simulink model "IEEE24bus"  (R2019b)
settings: Solver=VariableStepAuto  StartTime=0.0  StopTime=100  RelTol=1e-3
values from neighbouring files (symbols this model uses):
  C_b = 1/(w_b*Z_b)    (= 5.01433343075e-06)    [IEEE24_bus.m]
  Exc = [ 011	0	 200	0.02	1.12   0.5   0	0       0       0       0       0 ... (first row only)    [IEEE24_bus.m]
  G_data = [ 011	15.8 138	2.8	0.2     2.7	1.5     0.3     7.5     0.25	0.04	0.85	0.85	0.25	0.12	0 ... (first row only)    [IEEE24_bus.m]
  H011 = 4    [IEEE24_bus.m]
  H012 = 4    [IEEE24_bus.m]
  H013 = 4    [IEEE24_bus.m]
  H021 = 4    [IEEE24_bus.m]
  H022 = 4    [IEEE24_bus.m]
  H023 = 4    [IEEE24_bus.m]
  H024 = 4    [IEEE24_bus.m]
  H025 = 4    [IEEE24_bus.m]
  H026 = 4    [IEEE24_bus.m]
  H131 = 4    [IEEE24_bus.m]
  H132 = 4    [IEEE24_bus.m]
  H133 = 4    [IEEE24_bus.m]
  H134 = 4    [IEEE24_bus.m]
  H135 = 4    [IEEE24_bus.m]
  H151 = 4    [IEEE24_bus.m]
  H152 = 4    [IEEE24_bus.m]
  H153 = 4    [IEEE24_bus.m]
  H154 = 4    [IEEE24_bus.m]
  H161 = 4    [IEEE24_bus.m]
  H181 = 3.25    [IEEE24_bus.m]
  H211 = 4    [IEEE24_bus.m]
  H212 = 4    [IEEE24_bus.m]
  H213 = 4    [IEEE24_bus.m]
  H215 = 4    [IEEE24_bus.m]
  H216 = 4    [IEEE24_bus.m]
  H221 = 3.25    [IEEE24_bus.m]
  H231 = 4    [IEEE24_bus.m]
  H232 = 4    [IEEE24_bus.m]
  H233 = 4    [IEEE24_bus.m]
  H234 = 4    [IEEE24_bus.m]
  H235 = 4    [IEEE24_bus.m]
  L_b = Z_b/w_b    (= 1.40321608159)    [IEEE24_bus.m]
  PSSMODEL = 1    [IEEE24_bus.m]    (also in IEEE24bus_simplified_benchmark.m)
  Z_b = (V_b^2)/S_b    (= 529)    [IEEE24_bus.m]
undefined symbols (not defined in the file or in its folder): D1, Delta
libraries: powerlib x258, sps_avr x33, microgridLibrary x6
(part 2 of 6)

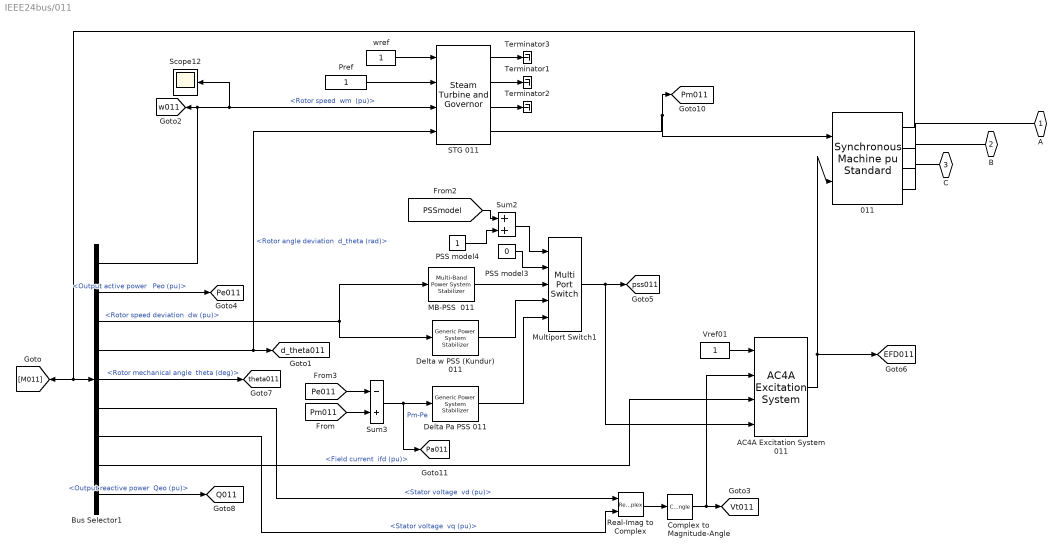
== system IEEE24bus/011 ==
  011 : powerlib/Machines/Synchronous Machine pu Standard  PresetModel=No  MechanicalLoad=Mechanical power Pm  ShowDetailedParameters=on  RotorType=Round  Units=per unit standard parameters  MeasurementBus=off  NominalParameters="[31.6*1E6  G_data(1,3)*1E3  60]"  Reactances1=[G_data(1,6),G_data(1,8),G_data(1,10),G_data(1,7),G_data(1,12),G_data(1,14),G_data(1,5)]  Reactances2=[G_data(6,6),G_data(6,8),G_data(6,10),G_data(6,7),G_data(6,12),G_data(6,14),G_data(6,5)]  dAxisTimeConstants=Open-circuit  qAxisTimeConstants=Open-circuit  TimeConstants1="[G_data(6,9)  G_data(6,11)  G_data(6,13)  G_data(6,15)]"  TimeConstants2="[G_data(1,9)  G_data(1,11)  G_data(1,13)  G_data(1,15)]"  TimeConstants3="[  5.9  0.033  0.023  ]"  TimeConstants4=[ 8.0, 0.03, 0.3371, 0.0295 ]  TimeConstants5=[ 1.01, 0.053, 0.1 ]  TimeConstants6=[ 1.3201, 0.023, 1.0, 0.07 ]  TimeConstants7="[  1.01  0.053  0.051266  ]"  TimeConstants8=[ 1.3201, 0.0231, 0.3371, 0.0295 ]  StatorResistance=0  Mechanical="[ H011 0  4 ]"  PolePairs=4  InitialConditions=[0 -49.0871 0.832503 0.832503 0.832503 -10.6328 -130.633 109.367 2.39024]  SetSaturation=off  Saturation=[0.6404,0.7127,0.8441,0.9214,0.9956,1.082,1.19,1.316,1.457;0.7,0.7698,0.8872,0.9466,0.9969,1.046,1.1,1.151,1.201]  LoadFlowParameters=[1 3330000000 20000 0 0]  TsPowergui=0  TsBlock=-1  IterativeModel=Forward Euler  IterativeDiscreteModel=Trapezoidal non iterative  BusType=PV  Pref=31.6*1e6  Qref=0  Qmin=-inf  Qmax=inf  PLF=0  QLF=0
      settings: SourceProductName=Simscape Power Systems
  AC4A Excitation System 011 : sps_avr/AC4A Excitation System  Tr=Exc(1,2)  KaTa="[Exc(1,3)   Exc(1,4)]"  VIminmax=[-10 10]  VRminmax=[-4.53 5.64]  TbTc="[Exc(1,5)  Exc(1,6)]"  Kc=0  v0=[1 2.3902]  TsBlock=0
      settings: SourceProductName=Simscape Power Systems  SourceProductBaseCode=PS
  Bus Selector1 : BusSelector  OutputSignals="Mechanical.Rotor speed  wm  (pu),Output active power   Peo (pu),Mechanical.Rotor speed deviation  dw (pu),Mechanical.Rotor angle deviation  d_theta (rad),Mechanical.Rotor mechanical angle  theta (deg),dq0 components.Stator voltage  vd (pu),dq0 components.Stator voltage  vq (pu),dq0 components.Field current  ifd (pu),Output reactive power  Qeo (pu)"
  Complex to Magnitude-Angle : ComplexToMagnitudeAngle  Output=Magnitude
  "Delta Pa PSS 011 " : powerlib/Machines/Generic Power System Stabilizer  Tsensor=15e-3  K=2.5*1.25  Twashout=1  Tleadlag1=[60e-3 1]  Tleadlag2=[0 0]  VSlimits=[-0.15 0.15]  Vinit=0  Plot_On=off  MagdB_On=on  FreqRange=logspace(-2,2,500)
      settings: SourceProductName=Simscape Power Systems  SourceProductBaseCode=PS
  "Delta w PSS (Kundur) 011 " : powerlib/Machines/Generic Power System Stabilizer  Tsensor=15e-3  K=30  Twashout=10  Tleadlag1=[50e-3 20e-3]  Tleadlag2=[3 5.4]  VSlimits=[-0.15 0.15]  Vinit=0  Plot_On=off  MagdB_On=on  FreqRange=logspace(-2,2,500)
      settings: SourceProductName=Simscape Power Systems  SourceProductBaseCode=PS
  MB-PSS  011 : powerlib/Machines/Multi-Band Power System Stabilizer  OperationMode=Simplified settings  Kg=1  GL=[0.1 10]  GI="[1  10]"  GH="[13  120]"  GLd=[66 66 9.4]  TcLF=[1.667 2 0 0 0 0 2 2.4 0 0 0 0 1 1]  GId=[66 66 47.6]  TcIF=[1 1 0.25 0.3 0 0 1 1 0.3 0.36 0 0 0 0]  GHd=[66 66 233]  TcHF="[0.01 0.012 0 0 0 0  0.012 0.0144 0 0 0 0 1 1]"  LIM=[.075 .15 .15 .15]  Plot_On=off  MagdB_On=off  FreqRange=logspace(-2,2,500)
      settings: SourceProductName=Simscape Power Systems  SourceProductBaseCode=PS
  Multiport Switch1 : MultiPortSwitch  Inputs=4  InputSameDT=on
  PSS model3 : Constant  Value=0
  PSS model4 : Constant
  Pref : Constant
  Real-Imag to Complex : RealImagToComplex
  STG 011 : powerlib/Machines/Steam Turbine and Governor  gentype=Tandem-compound (single mass)  reg1="[ 1  0.05    0 ]"  reg2="[ 0.001  0.15 ]"  reg3="[ -0.1  0.1  0  4.496 ]"  N=3600  turb1="[ 0  10   3.3   0.5   ]"  turb2="[   0   0.36    0.36   0.28   ]"  HA="[ 0.046  1.430  1.465   0.192 ]"  KA="[ 90.44  53.88  64.59   62.94  ]"  DA="[ 0.0115  0.3575  0.3663   0.0137  ]"  ini1=1  ini2=[0.779316,-31.4247]
      settings: SourceProductName=Simscape Power Systems  SourceProductBaseCode=PS
  Scope12 : Scope
  Sum2 : Sum  SaturateOnIntegerOverflow=on  InputSameDT=on  OutDataTypeStr=Inherit: Same as first input
  Sum3 : Sum  Inputs=-+  SaturateOnIntegerOverflow=on  InputSameDT=on  OutDataTypeStr=Inherit: Same as first input
  Terminator1 : Terminator
  Terminator2 : Terminator
  Terminator3 : Terminator
  Vref01 : Constant
  wref : Constant
  A : PMIOPort  Side=Left
  B : PMIOPort  Port=2  Side=Left
  C : PMIOPort  Port=3  Side=Left
  tag scope: EFD011=global, Pa011=global, Pe011=global, Pm011=global, Q011=global, Vt011=global, d_theta011=global, pss011=global, theta011=global, w011=global
  wires:
  Bus Selector1/7 -> Real-Imag to Complex/2  "<Stator voltage  vq (pu)>"
  Bus Selector1/6 -> Real-Imag to Complex/1  "<Stator voltage  vd (pu)>"
  wref/1 -> STG 011/1
  Vref01/1 -> AC4A Excitation System 011/1
  Bus Selector1/4 -> [d_theta011], STG 011/4  "<Rotor angle deviation  d_theta (rad)>"
  011/1 -> Bus Selector1/1, [M011]
  Bus Selector1/1 -> [w011], Scope12/1, STG 011/3  "<Rotor speed  wm  (pu)>"
  Bus Selector1/3 -> "Delta w PSS (Kundur) 011 "/1, MB-PSS  011/1  "<Rotor speed deviation  dw (pu)>"
  Real-Imag to Complex/1 -> Complex to Magnitude-Angle/1
  Complex to Magnitude-Angle/1 -> AC4A Excitation System 011/2, [Vt011]
  AC4A Excitation System 011/1 -> 011/2, [EFD011]
  Multiport Switch1/1 -> AC4A Excitation System 011/4, [pss011]
  Bus Selector1/5 -> [theta011]  "<Rotor mechanical angle  theta (deg)>"
  Bus Selector1/2 -> [Pe011]  "<Output active power   Peo (pu)>"
  Bus Selector1/8 -> AC4A Excitation System 011/3  "<Field current  ifd (pu)>"
  STG 011/4 -> [Pm011], 011/1
  Pref/1 -> STG 011/2
  Bus Selector1/9 -> [Q011]  "<Output reactive power  Qeo (pu)>"
  PSS model4/1 -> Sum2/2
  Sum2/1 -> Multiport Switch1/1
  [PSSmodel] -> Sum2/1
  PSS model3/1 -> Multiport Switch1/2
  Sum3/1 -> [Pa011], "Delta Pa PSS 011 "/1  "Pm-Pe"
  "Delta Pa PSS 011 "/1 -> Multiport Switch1/5
  "Delta w PSS (Kundur) 011 "/1 -> Multiport Switch1/4
  [Pm011] -> Sum3/2
  [Pe011] -> Sum3/1
  MB-PSS  011/1 -> Multiport Switch1/3
  STG 011/1 -> Terminator3/1
  STG 011/2 -> Terminator1/1
  STG 011/3 -> Terminator2/1
  connections:
  011/RConn1 -- A/RConn1
  011/RConn2 -- B/RConn1
  011/RConn3 -- C/RConn1

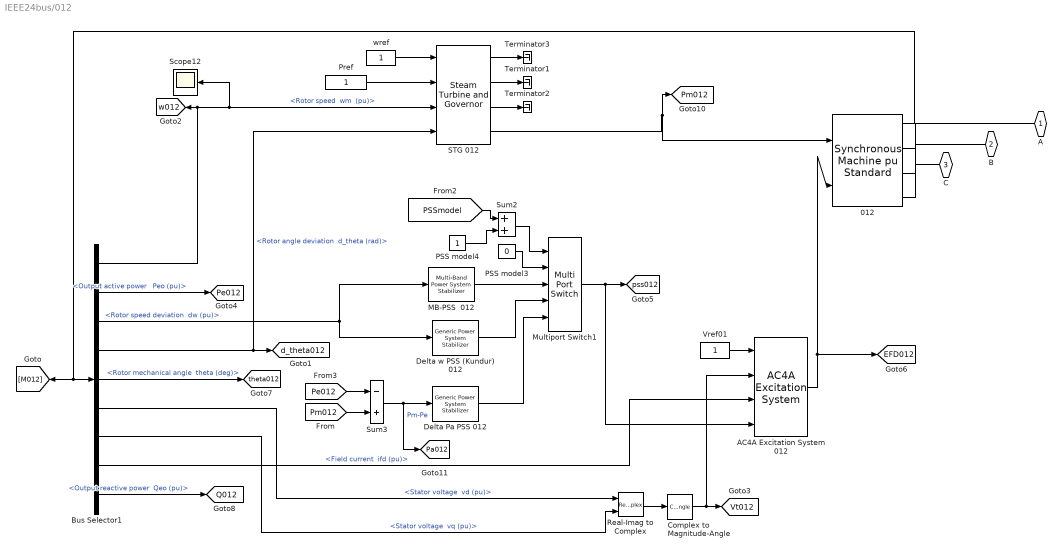
== system IEEE24bus/012 ==
  012 : powerlib/Machines/Synchronous Machine pu Standard  PresetModel=No  MechanicalLoad=Mechanical power Pm  ShowDetailedParameters=on  RotorType=Round  Units=per unit standard parameters  MeasurementBus=off  NominalParameters="[76*1E6  G_data(2,3)*1E3  60]"  Reactances1=[G_data(2,6),G_data(2,8),G_data(2,10),G_data(2,7),G_data(2,12),G_data(2,14),G_data(2,5)]  Reactances2=[G_data(6,6),G_data(6,8),G_data(6,10),G_data(6,7),G_data(6,12),G_data(6,14),G_data(6,5)]  dAxisTimeConstants=Open-circuit  qAxisTimeConstants=Open-circuit  TimeConstants1="[G_data(6,9)  G_data(6,11)  G_data(6,13)  G_data(6,15)]"  TimeConstants2="[G_data(2,9)  G_data(2,11)  G_data(2,13)  G_data(2,15)]"  TimeConstants3="[  5.9  0.033  0.023  ]"  TimeConstants4=[ 8.0, 0.03, 0.3371, 0.0295 ]  TimeConstants5=[ 1.01, 0.053, 0.1 ]  TimeConstants6=[ 1.3201, 0.023, 1.0, 0.07 ]  TimeConstants7="[  1.01  0.053  0.051266  ]"  TimeConstants8=[ 1.3201, 0.0231, 0.3371, 0.0295 ]  StatorResistance=0  Mechanical="[ H012 0  4 ]"  PolePairs=4  InitialConditions=[0 -49.0871 0.832503 0.832503 0.832503 -10.6328 -130.633 109.367 2.39024]  SetSaturation=off  Saturation=[0.6404,0.7127,0.8441,0.9214,0.9956,1.082,1.19,1.316,1.457;0.7,0.7698,0.8872,0.9466,0.9969,1.046,1.1,1.151,1.201]  LoadFlowParameters=[1 3330000000 20000 0 0]  TsPowergui=0  TsBlock=-1  IterativeModel=Forward Euler  IterativeDiscreteModel=Trapezoidal non iterative  BusType=PV  Pref=G_data(2,2)*1e6  Qref=0  Qmin=-inf  Qmax=inf  PLF=0  QLF=0
      settings: SourceProductName=Simscape Power Systems
  AC4A Excitation System 012 : sps_avr/AC4A Excitation System  Tr=Exc(2,2)  KaTa="[Exc(2,3)   Exc(2,4)]"  VIminmax=[-10 10]  VRminmax=[-4.53 5.64]  TbTc="[Exc(2,5)  Exc(2,6)]"  Kc=0  v0=[1 2.3902]  TsBlock=0
      settings: SourceProductName=Simscape Power Systems  SourceProductBaseCode=PS
  Bus Selector1 : BusSelector  OutputSignals="Mechanical.Rotor speed  wm  (pu),Output active power   Peo (pu),Mechanical.Rotor speed deviation  dw (pu),Mechanical.Rotor angle deviation  d_theta (rad),Mechanical.Rotor mechanical angle  theta (deg),dq0 components.Stator voltage  vd (pu),dq0 components.Stator voltage  vq (pu),dq0 components.Field current  ifd (pu),Output reactive power  Qeo (pu)"
  Complex to Magnitude-Angle : ComplexToMagnitudeAngle  Output=Magnitude
  "Delta Pa PSS 012 " : powerlib/Machines/Generic Power System Stabilizer  Tsensor=15e-3  K=2.5*1.25  Twashout=1  Tleadlag1=[60e-3 1]  Tleadlag2=[0 0]  VSlimits=[-0.15 0.15]  Vinit=0  Plot_On=off  MagdB_On=on  FreqRange=logspace(-2,2,500)
      settings: SourceProductName=Simscape Power Systems  SourceProductBaseCode=PS
  "Delta w PSS (Kundur) 012 " : powerlib/Machines/Generic Power System Stabilizer  Tsensor=15e-3  K=30  Twashout=10  Tleadlag1=[50e-3 20e-3]  Tleadlag2=[3 5.4]  VSlimits=[-0.15 0.15]  Vinit=0  Plot_On=off  MagdB_On=on  FreqRange=logspace(-2,2,500)
      settings: SourceProductName=Simscape Power Systems  SourceProductBaseCode=PS
  MB-PSS  012 : powerlib/Machines/Multi-Band Power System Stabilizer  OperationMode=Simplified settings  Kg=1  GL=[0.1 10]  GI="[1  10]"  GH="[13  120]"  GLd=[66 66 9.4]  TcLF=[1.667 2 0 0 0 0 2 2.4 0 0 0 0 1 1]  GId=[66 66 47.6]  TcIF=[1 1 0.25 0.3 0 0 1 1 0.3 0.36 0 0 0 0]  GHd=[66 66 233]  TcHF="[0.01 0.012 0 0 0 0  0.012 0.0144 0 0 0 0 1 1]"  LIM=[.075 .15 .15 .15]  Plot_On=off  MagdB_On=off  FreqRange=logspace(-2,2,500)
      settings: SourceProductName=Simscape Power Systems  SourceProductBaseCode=PS
  Multiport Switch1 : MultiPortSwitch  Inputs=4  InputSameDT=on
  PSS model3 : Constant  Value=0
  PSS model4 : Constant
  Pref : Constant
  Real-Imag to Complex : RealImagToComplex
  STG 012 : powerlib/Machines/Steam Turbine and Governor  gentype=Tandem-compound (single mass)  reg1="[ 1  0.05    0 ]"  reg2="[ 0.001  0.15 ]"  reg3="[ -0.1  0.1  0  4.496 ]"  N=3600  turb1="[ 0  10   3.3   0.5   ]"  turb2="[   0   0.36    0.36   0.28   ]"  HA="[ 0.046  1.430  1.465   0.192 ]"  KA="[ 90.44  53.88  64.59   62.94  ]"  DA="[ 0.0115  0.3575  0.3663   0.0137  ]"  ini1=0.2079  ini2=[0.779316,-31.4247]
      settings: SourceProductName=Simscape Power Systems  SourceProductBaseCode=PS
  Scope12 : Scope
  Sum2 : Sum  SaturateOnIntegerOverflow=on  InputSameDT=on  OutDataTypeStr=Inherit: Same as first input
  Sum3 : Sum  Inputs=-+  SaturateOnIntegerOverflow=on  InputSameDT=on  OutDataTypeStr=Inherit: Same as first input
  Terminator1 : Terminator
  Terminator2 : Terminator
  Terminator3 : Terminator
  Vref01 : Constant
  wref : Constant
  A : PMIOPort  Side=Left
  B : PMIOPort  Port=2  Side=Left
  C : PMIOPort  Port=3  Side=Left
  tag scope: EFD012=global, Pa012=global, Pe012=global, Pm012=global, Q012=global, Vt012=global, d_theta012=global, pss012=global, theta012=global, w012=global
  wires:
  Bus Selector1/7 -> Real-Imag to Complex/2  "<Stator voltage  vq (pu)>"
  Bus Selector1/6 -> Real-Imag to Complex/1  "<Stator voltage  vd (pu)>"
  wref/1 -> STG 012/1
  Vref01/1 -> AC4A Excitation System 012/1
  Bus Selector1/4 -> [d_theta012], STG 012/4  "<Rotor angle deviation  d_theta (rad)>"
  012/1 -> Bus Selector1/1, [M012]
  Bus Selector1/1 -> [w012], Scope12/1, STG 012/3  "<Rotor speed  wm  (pu)>"
  Bus Selector1/3 -> "Delta w PSS (Kundur) 012 "/1, MB-PSS  012/1  "<Rotor speed deviation  dw (pu)>"
  Real-Imag to Complex/1 -> Complex to Magnitude-Angle/1
  Complex to Magnitude-Angle/1 -> AC4A Excitation System 012/2, [Vt012]
  AC4A Excitation System 012/1 -> 012/2, [EFD012]
  Multiport Switch1/1 -> AC4A Excitation System 012/4, [pss012]
  Bus Selector1/5 -> [theta012]  "<Rotor mechanical angle  theta (deg)>"
  Bus Selector1/2 -> [Pe012]  "<Output active power   Peo (pu)>"
  Bus Selector1/8 -> AC4A Excitation System 012/3  "<Field current  ifd (pu)>"
  STG 012/4 -> [Pm012], 012/1
  Pref/1 -> STG 012/2
  Bus Selector1/9 -> [Q012]  "<Output reactive power  Qeo (pu)>"
  PSS model4/1 -> Sum2/2
  Sum2/1 -> Multiport Switch1/1
  [PSSmodel] -> Sum2/1
  PSS model3/1 -> Multiport Switch1/2
  Sum3/1 -> [Pa012], "Delta Pa PSS 012 "/1  "Pm-Pe"
  "Delta Pa PSS 012 "/1 -> Multiport Switch1/5
  "Delta w PSS (Kundur) 012 "/1 -> Multiport Switch1/4
  [Pm012] -> Sum3/2
  [Pe012] -> Sum3/1
  MB-PSS  012/1 -> Multiport Switch1/3
  STG 012/1 -> Terminator3/1
  STG 012/2 -> Terminator1/1
  STG 012/3 -> Terminator2/1
  connections:
  012/RConn1 -- A/RConn1
  012/RConn2 -- B/RConn1
  012/RConn3 -- C/RConn1

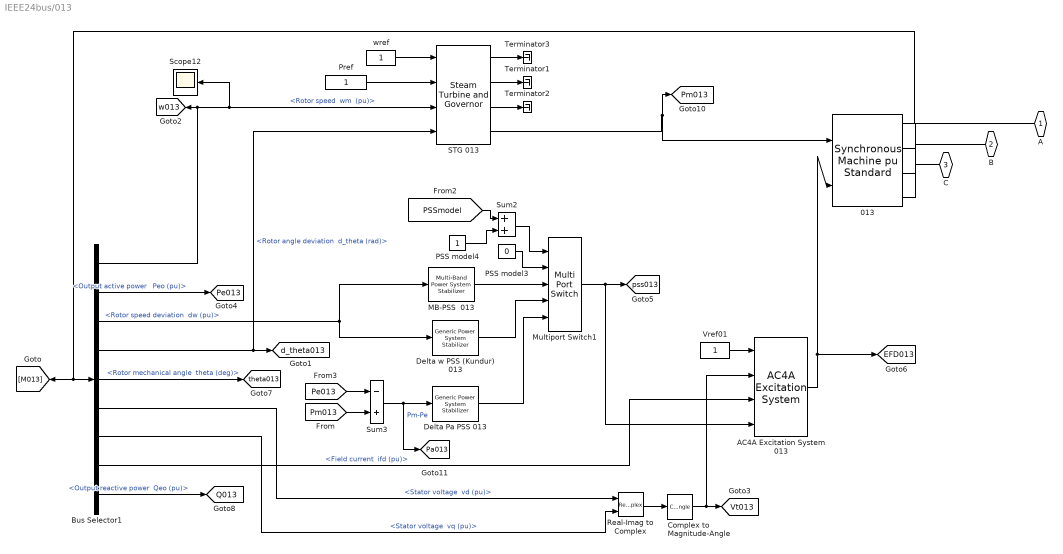
== system IEEE24bus/013 ==
  013 : powerlib/Machines/Synchronous Machine pu Standard  PresetModel=No  MechanicalLoad=Mechanical power Pm  ShowDetailedParameters=on  RotorType=Round  Units=per unit standard parameters  MeasurementBus=off  NominalParameters="[G_data(3,2)*1E6  G_data(3,3)*1E3  60]"  Reactances1=[G_data(3,6),G_data(3,8),G_data(3,10),G_data(3,7),G_data(3,12),G_data(3,14),G_data(3,5)]  Reactances2=[G_data(6,6),G_data(6,8),G_data(6,10),G_data(6,7),G_data(6,12),G_data(6,14),G_data(6,5)]  dAxisTimeConstants=Open-circuit  qAxisTimeConstants=Open-circuit  TimeConstants1="[G_data(6,9)  G_data(6,11)  G_data(6,13)  G_data(6,15)]"  TimeConstants2="[G_data(3,9)  G_data(3,11)  G_data(3,13)  G_data(3,15)]"  TimeConstants3="[  5.9  0.033  0.023  ]"  TimeConstants4=[ 8.0, 0.03, 0.3371, 0.0295 ]  TimeConstants5=[ 1.01, 0.053, 0.1 ]  TimeConstants6=[ 1.3201, 0.023, 1.0, 0.07 ]  TimeConstants7="[  1.01  0.053  0.051266  ]"  TimeConstants8=[ 1.3201, 0.0231, 0.3371, 0.0295 ]  StatorResistance=0  Mechanical="[ H013 0  4 ]"  PolePairs=4  InitialConditions=[0 -49.0871 0.832503 0.832503 0.832503 -10.6328 -130.633 109.367 2.39024]  SetSaturation=off  Saturation=[0.6404,0.7127,0.8441,0.9214,0.9956,1.082,1.19,1.316,1.457;0.7,0.7698,0.8872,0.9466,0.9969,1.046,1.1,1.151,1.201]  LoadFlowParameters=[1 3330000000 20000 0 0]  TsPowergui=0  TsBlock=-1  IterativeModel=Forward Euler  IterativeDiscreteModel=Trapezoidal non iterative  BusType=PV  Pref=G_data(3,2)*1e6  Qref=0  Qmin=-inf  Qmax=inf  PLF=0  QLF=0
      settings: SourceProductName=Simscape Power Systems
  AC4A Excitation System 013 : sps_avr/AC4A Excitation System  Tr=Exc(3,2)  KaTa="[Exc(3,3)   Exc(3,4)]"  VIminmax=[-10 10]  VRminmax=[-4.53 5.64]  TbTc="[Exc(3,5)  Exc(3,6)]"  Kc=0  v0=[1 2.3902]  TsBlock=0
      settings: SourceProductName=Simscape Power Systems  SourceProductBaseCode=PS
  Bus Selector1 : BusSelector  OutputSignals="Mechanical.Rotor speed  wm  (pu),Output active power   Peo (pu),Mechanical.Rotor speed deviation  dw (pu),Mechanical.Rotor angle deviation  d_theta (rad),Mechanical.Rotor mechanical angle  theta (deg),dq0 components.Stator voltage  vd (pu),dq0 components.Stator voltage  vq (pu),dq0 components.Field current  ifd (pu),Output reactive power  Qeo (pu)"
  Complex to Magnitude-Angle : ComplexToMagnitudeAngle  Output=Magnitude
  "Delta Pa PSS 013 " : powerlib/Machines/Generic Power System Stabilizer  Tsensor=15e-3  K=2.5*1.25  Twashout=1  Tleadlag1=[60e-3 1]  Tleadlag2=[0 0]  VSlimits=[-0.15 0.15]  Vinit=0  Plot_On=off  MagdB_On=on  FreqRange=logspace(-2,2,500)
      settings: SourceProductName=Simscape Power Systems  SourceProductBaseCode=PS
  "Delta w PSS (Kundur) 013 " : powerlib/Machines/Generic Power System Stabilizer  Tsensor=15e-3  K=30  Twashout=10  Tleadlag1=[50e-3 20e-3]  Tleadlag2=[3 5.4]  VSlimits=[-0.15 0.15]  Vinit=0  Plot_On=off  MagdB_On=on  FreqRange=logspace(-2,2,500)
      settings: SourceProductName=Simscape Power Systems  SourceProductBaseCode=PS
  MB-PSS  013 : powerlib/Machines/Multi-Band Power System Stabilizer  OperationMode=Simplified settings  Kg=1  GL=[0.1 10]  GI="[1  10]"  GH="[13  120]"  GLd=[66 66 9.4]  TcLF=[1.667 2 0 0 0 0 2 2.4 0 0 0 0 1 1]  GId=[66 66 47.6]  TcIF=[1 1 0.25 0.3 0 0 1 1 0.3 0.36 0 0 0 0]  GHd=[66 66 233]  TcHF="[0.01 0.012 0 0 0 0  0.012 0.0144 0 0 0 0 1 1]"  LIM=[.075 .15 .15 .15]  Plot_On=off  MagdB_On=off  FreqRange=logspace(-2,2,500)
      settings: SourceProductName=Simscape Power Systems  SourceProductBaseCode=PS
  Multiport Switch1 : MultiPortSwitch  Inputs=4  InputSameDT=on
  PSS model3 : Constant  Value=0
  PSS model4 : Constant
  Pref : Constant
  Real-Imag to Complex : RealImagToComplex
  STG 013 : powerlib/Machines/Steam Turbine and Governor  gentype=Tandem-compound (single mass)  reg1="[ 1  0.05    0 ]"  reg2="[ 0.001  0.15 ]"  reg3="[ -0.1  0.1  0  4.496 ]"  N=3600  turb1="[ 0  10   3.3   0.5   ]"  turb2="[   0   0.36    0.36   0.28   ]"  HA="[ 0.046  1.430  1.465   0.192 ]"  KA="[ 90.44  53.88  64.59   62.94  ]"  DA="[ 0.0115  0.3575  0.3663   0.0137  ]"  ini1=0.9  ini2=[0.779316,-31.4247]
      settings: SourceProductName=Simscape Power Systems  SourceProductBaseCode=PS
  Scope12 : Scope
  Sum2 : Sum  SaturateOnIntegerOverflow=on  InputSameDT=on  OutDataTypeStr=Inherit: Same as first input
  Sum3 : Sum  Inputs=-+  SaturateOnIntegerOverflow=on  InputSameDT=on  OutDataTypeStr=Inherit: Same as first input
  Terminator1 : Terminator
  Terminator2 : Terminator
  Terminator3 : Terminator
  Vref01 : Constant
  wref : Constant
  A : PMIOPort  Side=Left
  B : PMIOPort  Port=2  Side=Left
  C : PMIOPort  Port=3  Side=Left
  tag scope: EFD013=global, Pa013=global, Pe013=global, Pm013=global, Q013=global, Vt013=global, d_theta013=global, pss013=global, theta013=global, w013=global
  wires:
  Bus Selector1/7 -> Real-Imag to Complex/2  "<Stator voltage  vq (pu)>"
  Bus Selector1/6 -> Real-Imag to Complex/1  "<Stator voltage  vd (pu)>"
  wref/1 -> STG 013/1
  Vref01/1 -> AC4A Excitation System 013/1
  Bus Selector1/4 -> [d_theta013], STG 013/4  "<Rotor angle deviation  d_theta (rad)>"
  013/1 -> Bus Selector1/1, [M013]
  Bus Selector1/1 -> [w013], Scope12/1, STG 013/3  "<Rotor speed  wm  (pu)>"
  Bus Selector1/3 -> "Delta w PSS (Kundur) 013 "/1, MB-PSS  013/1  "<Rotor speed deviation  dw (pu)>"
  Real-Imag to Complex/1 -> Complex to Magnitude-Angle/1
  Complex to Magnitude-Angle/1 -> AC4A Excitation System 013/2, [Vt013]
  AC4A Excitation System 013/1 -> 013/2, [EFD013]
  Multiport Switch1/1 -> AC4A Excitation System 013/4, [pss013]
  Bus Selector1/5 -> [theta013]  "<Rotor mechanical angle  theta (deg)>"
  Bus Selector1/2 -> [Pe013]  "<Output active power   Peo (pu)>"
  Bus Selector1/8 -> AC4A Excitation System 013/3  "<Field current  ifd (pu)>"
  STG 013/4 -> [Pm013], 013/1
  Pref/1 -> STG 013/2
  Bus Selector1/9 -> [Q013]  "<Output reactive power  Qeo (pu)>"
  PSS model4/1 -> Sum2/2
  Sum2/1 -> Multiport Switch1/1
  [PSSmodel] -> Sum2/1
  PSS model3/1 -> Multiport Switch1/2
  Sum3/1 -> [Pa013], "Delta Pa PSS 013 "/1  "Pm-Pe"
  "Delta Pa PSS 013 "/1 -> Multiport Switch1/5
  "Delta w PSS (Kundur) 013 "/1 -> Multiport Switch1/4
  [Pm013] -> Sum3/2
  [Pe013] -> Sum3/1
  MB-PSS  013/1 -> Multiport Switch1/3
  STG 013/1 -> Terminator3/1
  STG 013/2 -> Terminator1/1
  STG 013/3 -> Terminator2/1
  connections:
  013/RConn1 -- A/RConn1
  013/RConn2 -- B/RConn1
  013/RConn3 -- C/RConn1

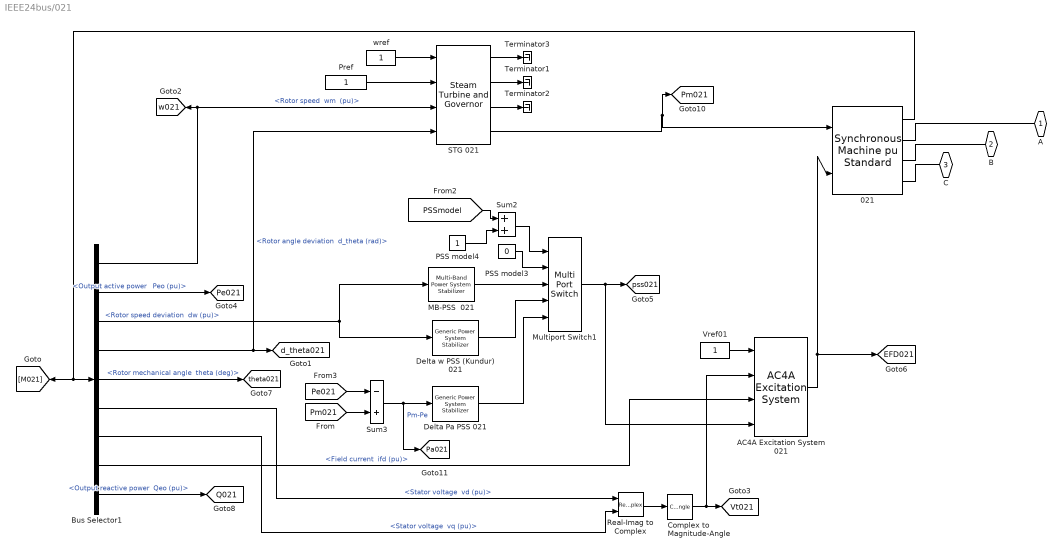
== system IEEE24bus/021  ==
  021 : powerlib/Machines/Synchronous Machine pu Standard  PresetModel=No  MechanicalLoad=Mechanical power Pm  ShowDetailedParameters=on  RotorType=Round  Units=per unit standard parameters  MeasurementBus=off  NominalParameters="[40*1E6  G_data(4,3)*1E3  60]"  Reactances1=[G_data(4,6),G_data(4,8),G_data(4,10),G_data(4,7),G_data(4,12),G_data(4,14),G_data(4,5)]  Reactances2=[G_data(6,6),G_data(6,8),G_data(6,10),G_data(6,7),G_data(6,12),G_data(6,14),G_data(6,5)]  dAxisTimeConstants=Open-circuit  qAxisTimeConstants=Open-circuit  TimeConstants1="[G_data(6,9)  G_data(6,11)  G_data(6,13)  G_data(6,15)]"  TimeConstants2="[G_data(4,9)  G_data(4,11)  G_data(4,13)  G_data(4,15)]"  TimeConstants3="[  5.9  0.033  0.023  ]"  TimeConstants4=[ 8.0, 0.03, 0.3371, 0.0295 ]  TimeConstants5=[ 1.01, 0.053, 0.1 ]  TimeConstants6=[ 1.3201, 0.023, 1.0, 0.07 ]  TimeConstants7="[  1.01  0.053  0.051266  ]"  TimeConstants8=[ 1.3201, 0.0231, 0.3371, 0.0295 ]  StatorResistance=0  Mechanical="[ H021 0  4 ]"  PolePairs=4  InitialConditions=[0 -49.0871 0.832503 0.832503 0.832503 -10.6328 -130.633 109.367 2.39024]  SetSaturation=off  Saturation=[0.6404,0.7127,0.8441,0.9214,0.9956,1.082,1.19,1.316,1.457;0.7,0.7698,0.8872,0.9466,0.9969,1.046,1.1,1.151,1.201]  LoadFlowParameters=[1 3330000000 20000 0 0]  TsPowergui=0  TsBlock=-1  IterativeModel=Forward Euler  IterativeDiscreteModel=Trapezoidal non iterative  BusType=PV  Pref=40*1e6  Qref=0  Qmin=-inf  Qmax=inf  PLF=0  QLF=0
      settings: SourceProductName=Simscape Power Systems
  AC4A Excitation System 021 : sps_avr/AC4A Excitation System  Tr=Exc(1,2)  KaTa="[Exc(1,3)   Exc(1,4)]"  VIminmax=[-10 10]  VRminmax=[-4.53 5.64]  TbTc="[Exc(1,5)  Exc(1,6)]"  Kc=0  v0=[1 2.3902]  TsBlock=0
      settings: SourceProductName=Simscape Power Systems  SourceProductBaseCode=PS
  Bus Selector1 : BusSelector  OutputSignals="Mechanical.Rotor speed  wm  (pu),Output active power   Peo (pu),Mechanical.Rotor speed deviation  dw (pu),Mechanical.Rotor angle deviation  d_theta (rad),Mechanical.Rotor mechanical angle  theta (deg),dq0 components.Stator voltage  vd (pu),dq0 components.Stator voltage  vq (pu),dq0 components.Field current  ifd (pu),Output reactive power  Qeo (pu)"
  Complex to Magnitude-Angle : ComplexToMagnitudeAngle  Output=Magnitude
  "Delta Pa PSS 021 " : powerlib/Machines/Generic Power System Stabilizer  Tsensor=15e-3  K=2.5*1.25  Twashout=1  Tleadlag1=[60e-3 1]  Tleadlag2=[0 0]  VSlimits=[-0.15 0.15]  Vinit=0  Plot_On=off  MagdB_On=on  FreqRange=logspace(-2,2,500)
      settings: SourceProductName=Simscape Power Systems  SourceProductBaseCode=PS
  "Delta w PSS (Kundur) 021 " : powerlib/Machines/Generic Power System Stabilizer  Tsensor=15e-3  K=30  Twashout=10  Tleadlag1=[50e-3 20e-3]  Tleadlag2=[3 5.4]  VSlimits=[-0.15 0.15]  Vinit=0  Plot_On=off  MagdB_On=on  FreqRange=logspace(-2,2,500)
      settings: SourceProductName=Simscape Power Systems  SourceProductBaseCode=PS
  MB-PSS  021 : powerlib/Machines/Multi-Band Power System Stabilizer  OperationMode=Simplified settings  Kg=1  GL=[0.1 10]  GI="[1  10]"  GH="[13  120]"  GLd=[66 66 9.4]  TcLF=[1.667 2 0 0 0 0 2 2.4 0 0 0 0 1 1]  GId=[66 66 47.6]  TcIF=[1 1 0.25 0.3 0 0 1 1 0.3 0.36 0 0 0 0]  GHd=[66 66 233]  TcHF="[0.01 0.012 0 0 0 0  0.012 0.0144 0 0 0 0 1 1]"  LIM=[.075 .15 .15 .15]  Plot_On=off  MagdB_On=off  FreqRange=logspace(-2,2,500)
      settings: SourceProductName=Simscape Power Systems  SourceProductBaseCode=PS
  Multiport Switch1 : MultiPortSwitch  Inputs=4  InputSameDT=on
  PSS model3 : Constant  Value=0
  PSS model4 : Constant
  Pref : Constant
  Real-Imag to Complex : RealImagToComplex
  STG 021 : powerlib/Machines/Steam Turbine and Governor  gentype=Tandem-compound (single mass)  reg1="[ 1  0.05    0 ]"  reg2="[ 0.001  0.15 ]"  reg3="[ -0.1  0.1  0  4.496 ]"  N=3600  turb1="[ 0  10   3.3   0.5   ]"  turb2="[   0   0.36    0.36   0.28   ]"  HA="[ 0.046  1.430  1.465   0.192 ]"  KA="[ 90.44  53.88  64.59   62.94  ]"  DA="[ 0.0115  0.3575  0.3663   0.0137  ]"  ini1=0.98  ini2=[0.779316,-31.4247]
      settings: SourceProductName=Simscape Power Systems  SourceProductBaseCode=PS
  Sum2 : Sum  SaturateOnIntegerOverflow=on  InputSameDT=on  OutDataTypeStr=Inherit: Same as first input
  Sum3 : Sum  Inputs=-+  SaturateOnIntegerOverflow=on  InputSameDT=on  OutDataTypeStr=Inherit: Same as first input
  Terminator1 : Terminator
  Terminator2 : Terminator
  Terminator3 : Terminator
  Vref01 : Constant
  wref : Constant
  A : PMIOPort  Side=Left
  B : PMIOPort  Port=2  Side=Left
  C : PMIOPort  Port=3  Side=Left
  tag scope: EFD021=global, Pa021=global, Pe021=global, Pm021=global, Q021=global, Vt021=global, d_theta021=global, pss021=global, theta021=global, w021=global
  wires:
  Bus Selector1/7 -> Real-Imag to Complex/2  "<Stator voltage  vq (pu)>"
  Bus Selector1/6 -> Real-Imag to Complex/1  "<Stator voltage  vd (pu)>"
  wref/1 -> STG 021/1
  Vref01/1 -> AC4A Excitation System 021/1
  Bus Selector1/4 -> [d_theta021], STG 021/4  "<Rotor angle deviation  d_theta (rad)>"
  021/1 -> Bus Selector1/1, [M021]
  Bus Selector1/1 -> [w021], STG 021/3  "<Rotor speed  wm  (pu)>"
  Bus Selector1/3 -> "Delta w PSS (Kundur) 021 "/1, MB-PSS  021/1  "<Rotor speed deviation  dw (pu)>"
  Real-Imag to Complex/1 -> Complex to Magnitude-Angle/1
  Complex to Magnitude-Angle/1 -> AC4A Excitation System 021/2, [Vt021]
  AC4A Excitation System 021/1 -> 021/2, [EFD021]
  Multiport Switch1/1 -> AC4A Excitation System 021/4, [pss021]
  Bus Selector1/5 -> [theta021]  "<Rotor mechanical angle  theta (deg)>"
  Bus Selector1/2 -> [Pe021]  "<Output active power   Peo (pu)>"
  Bus Selector1/8 -> AC4A Excitation System 021/3  "<Field current  ifd (pu)>"
  STG 021/4 -> [Pm021], 021/1
  Pref/1 -> STG 021/2
  Bus Selector1/9 -> [Q021]  "<Output reactive power  Qeo (pu)>"
  PSS model4/1 -> Sum2/2
  Sum2/1 -> Multiport Switch1/1
  [PSSmodel] -> Sum2/1
  PSS model3/1 -> Multiport Switch1/2
  Sum3/1 -> [Pa021], "Delta Pa PSS 021 "/1  "Pm-Pe"
  "Delta Pa PSS 021 "/1 -> Multiport Switch1/5
  "Delta w PSS (Kundur) 021 "/1 -> Multiport Switch1/4
  [Pm021] -> Sum3/2
  [Pe021] -> Sum3/1
  MB-PSS  021/1 -> Multiport Switch1/3
  STG 021/1 -> Terminator3/1
  STG 021/2 -> Terminator1/1
  STG 021/3 -> Terminator2/1
  connections:
  021/RConn1 -- A/RConn1
  021/RConn2 -- B/RConn1
  021/RConn3 -- C/RConn1

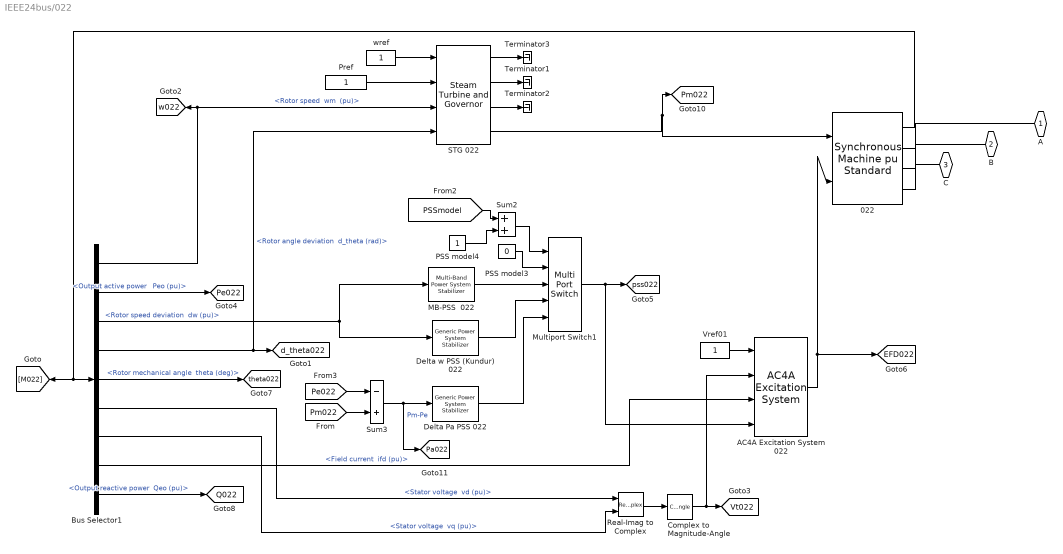
== system IEEE24bus/022 ==
  022 : powerlib/Machines/Synchronous Machine pu Standard  PresetModel=No  MechanicalLoad=Mechanical power Pm  ShowDetailedParameters=on  RotorType=Round  Units=per unit standard parameters  MeasurementBus=off  NominalParameters="[G_data(5,2)*1E6  G_data(5,3)*1E3  60]"  Reactances1=[G_data(5,6),G_data(5,8),G_data(5,10),G_data(5,7),G_data(5,12),G_data(5,14),G_data(5,5)]  Reactances2=[G_data(6,6),G_data(6,8),G_data(6,10),G_data(6,7),G_data(6,12),G_data(6,14),G_data(6,5)]  dAxisTimeConstants=Open-circuit  qAxisTimeConstants=Open-circuit  TimeConstants1="[G_data(6,9)  G_data(6,11)  G_data(6,13)  G_data(6,15)]"  TimeConstants2="[G_data(5,9)  G_data(5,11)  G_data(5,13)  G_data(5,15)]"  TimeConstants3="[  5.9  0.033  0.023  ]"  TimeConstants4=[ 8.0, 0.03, 0.3371, 0.0295 ]  TimeConstants5=[ 1.01, 0.053, 0.1 ]  TimeConstants6=[ 1.3201, 0.023, 1.0, 0.07 ]  TimeConstants7="[  1.01  0.053  0.051266  ]"  TimeConstants8=[ 1.3201, 0.0231, 0.3371, 0.0295 ]  StatorResistance=0  Mechanical="[ H022 0  4 ]"  PolePairs=4  InitialConditions=[0 -49.0871 0.832503 0.832503 0.832503 -10.6328 -130.633 109.367 2.39024]  SetSaturation=off  Saturation=[0.6404,0.7127,0.8441,0.9214,0.9956,1.082,1.19,1.316,1.457;0.7,0.7698,0.8872,0.9466,0.9969,1.046,1.1,1.151,1.201]  LoadFlowParameters=[1 3330000000 20000 0 0]  TsPowergui=0  TsBlock=-1  IterativeModel=Forward Euler  IterativeDiscreteModel=Trapezoidal non iterative  BusType=PV  Pref=G_data(5,2)*1e6  Qref=0  Qmin=-inf  Qmax=inf  PLF=0  QLF=0
      settings: SourceProductName=Simscape Power Systems
  AC4A Excitation System 022 : sps_avr/AC4A Excitation System  Tr=Exc(1,2)  KaTa="[Exc(1,3)   Exc(1,4)]"  VIminmax=[-10 10]  VRminmax=[-4.53 5.64]  TbTc="[Exc(1,5)  Exc(1,6)]"  Kc=0  v0=[1 2.3902]  TsBlock=0
      settings: SourceProductName=Simscape Power Systems  SourceProductBaseCode=PS
  Bus Selector1 : BusSelector  OutputSignals="Mechanical.Rotor speed  wm  (pu),Output active power   Peo (pu),Mechanical.Rotor speed deviation  dw (pu),Mechanical.Rotor angle deviation  d_theta (rad),Mechanical.Rotor mechanical angle  theta (deg),dq0 components.Stator voltage  vd (pu),dq0 components.Stator voltage  vq (pu),dq0 components.Field current  ifd (pu),Output reactive power  Qeo (pu)"
  Complex to Magnitude-Angle : ComplexToMagnitudeAngle  Output=Magnitude
  "Delta Pa PSS 022 " : powerlib/Machines/Generic Power System Stabilizer  Tsensor=15e-3  K=2.5*1.25  Twashout=1  Tleadlag1=[60e-3 1]  Tleadlag2=[0 0]  VSlimits=[-0.15 0.15]  Vinit=0  Plot_On=off  MagdB_On=on  FreqRange=logspace(-2,2,500)
      settings: SourceProductName=Simscape Power Systems  SourceProductBaseCode=PS
  "Delta w PSS (Kundur) 022 " : powerlib/Machines/Generic Power System Stabilizer  Tsensor=15e-3  K=30  Twashout=10  Tleadlag1=[50e-3 20e-3]  Tleadlag2=[3 5.4]  VSlimits=[-0.15 0.15]  Vinit=0  Plot_On=off  MagdB_On=on  FreqRange=logspace(-2,2,500)
      settings: SourceProductName=Simscape Power Systems  SourceProductBaseCode=PS
  MB-PSS  022 : powerlib/Machines/Multi-Band Power System Stabilizer  OperationMode=Simplified settings  Kg=1  GL=[0.1 10]  GI="[1  10]"  GH="[13  120]"  GLd=[66 66 9.4]  TcLF=[1.667 2 0 0 0 0 2 2.4 0 0 0 0 1 1]  GId=[66 66 47.6]  TcIF=[1 1 0.25 0.3 0 0 1 1 0.3 0.36 0 0 0 0]  GHd=[66 66 233]  TcHF="[0.01 0.012 0 0 0 0  0.012 0.0144 0 0 0 0 1 1]"  LIM=[.075 .15 .15 .15]  Plot_On=off  MagdB_On=off  FreqRange=logspace(-2,2,500)
      settings: SourceProductName=Simscape Power Systems  SourceProductBaseCode=PS
  Multiport Switch1 : MultiPortSwitch  Inputs=4  InputSameDT=on
  PSS model3 : Constant  Value=0
  PSS model4 : Constant
  Pref : Constant
  Real-Imag to Complex : RealImagToComplex
  STG 022 : powerlib/Machines/Steam Turbine and Governor  gentype=Tandem-compound (single mass)  reg1="[ 1  0.05    0 ]"  reg2="[ 0.001  0.15 ]"  reg3="[ -0.1  0.1  0  4.496 ]"  N=3600  turb1="[ 0  10   3.3   0.5   ]"  turb2="[   0   0.36    0.36   0.28   ]"  HA="[ 0.046  1.430  1.465   0.192 ]"  KA="[ 90.44  53.88  64.59   62.94  ]"  DA="[ 0.0115  0.3575  0.3663   0.0137  ]"  ini1=1  ini2=[0.779316,-31.4247]
      settings: SourceProductName=Simscape Power Systems  SourceProductBaseCode=PS
  Sum2 : Sum  SaturateOnIntegerOverflow=on  InputSameDT=on  OutDataTypeStr=Inherit: Same as first input
  Sum3 : Sum  Inputs=-+  SaturateOnIntegerOverflow=on  InputSameDT=on  OutDataTypeStr=Inherit: Same as first input
  Terminator1 : Terminator
  Terminator2 : Terminator
  Terminator3 : Terminator
  Vref01 : Constant
  wref : Constant
  A : PMIOPort  Side=Left
  B : PMIOPort  Port=2  Side=Left
  C : PMIOPort  Port=3  Side=Left
  tag scope: EFD022=global, Pa022=global, Pe022=global, Pm022=global, Q022=global, Vt022=global, d_theta022=global, pss022=global, theta022=global, w022=global
  wires:
  Bus Selector1/7 -> Real-Imag to Complex/2  "<Stator voltage  vq (pu)>"
  Bus Selector1/6 -> Real-Imag to Complex/1  "<Stator voltage  vd (pu)>"
  wref/1 -> STG 022/1
  Vref01/1 -> AC4A Excitation System 022/1
  Bus Selector1/4 -> [d_theta022], STG 022/4  "<Rotor angle deviation  d_theta (rad)>"
  022/1 -> Bus Selector1/1, [M022]
  Bus Selector1/1 -> [w022], STG 022/3  "<Rotor speed  wm  (pu)>"
  Bus Selector1/3 -> "Delta w PSS (Kundur) 022 "/1, MB-PSS  022/1  "<Rotor speed deviation  dw (pu)>"
  Real-Imag to Complex/1 -> Complex to Magnitude-Angle/1
  Complex to Magnitude-Angle/1 -> AC4A Excitation System 022/2, [Vt022]
  AC4A Excitation System 022/1 -> 022/2, [EFD022]
  Multiport Switch1/1 -> AC4A Excitation System 022/4, [pss022]
  Bus Selector1/5 -> [theta022]  "<Rotor mechanical angle  theta (deg)>"
  Bus Selector1/2 -> [Pe022]  "<Output active power   Peo (pu)>"
  Bus Selector1/8 -> AC4A Excitation System 022/3  "<Field current  ifd (pu)>"
  STG 022/4 -> [Pm022], 022/1
  Pref/1 -> STG 022/2
  Bus Selector1/9 -> [Q022]  "<Output reactive power  Qeo (pu)>"
  PSS model4/1 -> Sum2/2
  Sum2/1 -> Multiport Switch1/1
  [PSSmodel] -> Sum2/1
  PSS model3/1 -> Multiport Switch1/2
  Sum3/1 -> [Pa022], "Delta Pa PSS 022 "/1  "Pm-Pe"
  "Delta Pa PSS 022 "/1 -> Multiport Switch1/5
  "Delta w PSS (Kundur) 022 "/1 -> Multiport Switch1/4
  [Pm022] -> Sum3/2
  [Pe022] -> Sum3/1
  MB-PSS  022/1 -> Multiport Switch1/3
  STG 022/1 -> Terminator3/1
  STG 022/2 -> Terminator1/1
  STG 022/3 -> Terminator2/1
  connections:
  022/RConn1 -- A/RConn1
  022/RConn2 -- B/RConn1
  022/RConn3 -- C/RConn1

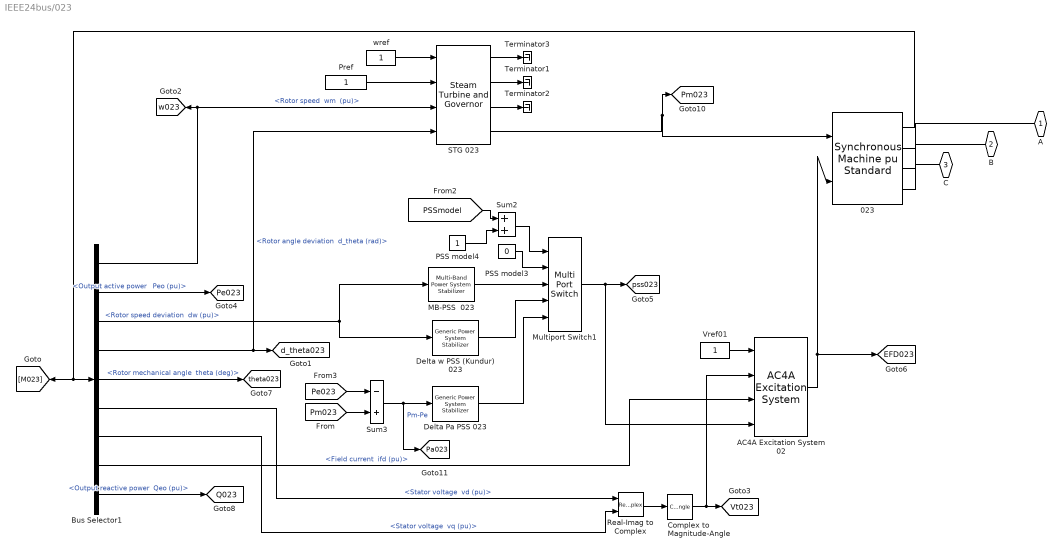
== system IEEE24bus/023 ==
  023 : powerlib/Machines/Synchronous Machine pu Standard  PresetModel=No  MechanicalLoad=Mechanical power Pm  ShowDetailedParameters=on  RotorType=Round  Units=per unit standard parameters  MeasurementBus=off  NominalParameters="[300*1E6  G_data(6,3)*1E3  60]"  Reactances1=[G_data(6,6),G_data(6,8),G_data(6,10),G_data(6,7),G_data(6,12),G_data(6,14),G_data(6,5)]  Reactances2=[G_data(6,6),G_data(6,8),G_data(6,10),G_data(6,7),G_data(6,12),G_data(6,14),G_data(6,5)]  dAxisTimeConstants=Open-circuit  qAxisTimeConstants=Open-circuit  TimeConstants1="[G_data(6,9)  G_data(6,11)  G_data(6,13)  G_data(6,15)]"  TimeConstants2="[G_data(6,9)  G_data(6,11)  G_data(6,13)  G_data(6,15)]"  TimeConstants3="[  5.9  0.033  0.023  ]"  TimeConstants4=[ 8.0, 0.03, 0.3371, 0.0295 ]  TimeConstants5=[ 1.01, 0.053, 0.1 ]  TimeConstants6=[ 1.3201, 0.023, 1.0, 0.07 ]  TimeConstants7="[  1.01  0.053  0.051266  ]"  TimeConstants8=[ 1.3201, 0.0231, 0.3371, 0.0295 ]  StatorResistance=0  Mechanical="[ H023 0  4 ]"  PolePairs=4  InitialConditions=[0 -49.0871 0.832503 0.832503 0.832503 -10.6328 -130.633 109.367 2.39024]  SetSaturation=off  Saturation=[0.6404,0.7127,0.8441,0.9214,0.9956,1.082,1.19,1.316,1.457;0.7,0.7698,0.8872,0.9466,0.9969,1.046,1.1,1.151,1.201]  LoadFlowParameters=[1 3330000000 20000 0 0]  TsPowergui=0  TsBlock=-1  IterativeModel=Forward Euler  IterativeDiscreteModel=Trapezoidal non iterative  BusType=PV  Pref=300*1e6  Qref=0  Qmin=-inf  Qmax=inf  PLF=0  QLF=0
      settings: SourceProductName=Simscape Power Systems
  AC4A Excitation System 02 : sps_avr/AC4A Excitation System  Tr=Exc(6,2)  KaTa="[Exc(6,3)   Exc(6,4)]"  VIminmax=[-10 10]  VRminmax=[-4.53 5.64]  TbTc="[Exc(6,5)  Exc(6,6)]"  Kc=0  v0=[1 2.3902]  TsBlock=0
      settings: SourceProductName=Simscape Power Systems  SourceProductBaseCode=PS
  Bus Selector1 : BusSelector  OutputSignals="Mechanical.Rotor speed  wm  (pu),Output active power   Peo (pu),Mechanical.Rotor speed deviation  dw (pu),Mechanical.Rotor angle deviation  d_theta (rad),Mechanical.Rotor mechanical angle  theta (deg),dq0 components.Stator voltage  vd (pu),dq0 components.Stator voltage  vq (pu),dq0 components.Field current  ifd (pu),Output reactive power  Qeo (pu)"
  Complex to Magnitude-Angle : ComplexToMagnitudeAngle  Output=Magnitude
  "Delta Pa PSS 023 " : powerlib/Machines/Generic Power System Stabilizer  Tsensor=15e-3  K=2.5*1.25  Twashout=1  Tleadlag1=[60e-3 1]  Tleadlag2=[0 0]  VSlimits=[-0.15 0.15]  Vinit=0  Plot_On=off  MagdB_On=on  FreqRange=logspace(-2,2,500)
      settings: SourceProductName=Simscape Power Systems  SourceProductBaseCode=PS
  "Delta w PSS (Kundur) 023 " : powerlib/Machines/Generic Power System Stabilizer  Tsensor=15e-3  K=30  Twashout=10  Tleadlag1=[50e-3 20e-3]  Tleadlag2=[3 5.4]  VSlimits=[-0.15 0.15]  Vinit=0  Plot_On=off  MagdB_On=on  FreqRange=logspace(-2,2,500)
      settings: SourceProductName=Simscape Power Systems  SourceProductBaseCode=PS
  MB-PSS  023 : powerlib/Machines/Multi-Band Power System Stabilizer  OperationMode=Simplified settings  Kg=1  GL=[0.1 10]  GI="[1  10]"  GH="[13  120]"  GLd=[66 66 9.4]  TcLF=[1.667 2 0 0 0 0 2 2.4 0 0 0 0 1 1]  GId=[66 66 47.6]  TcIF=[1 1 0.25 0.3 0 0 1 1 0.3 0.36 0 0 0 0]  GHd=[66 66 233]  TcHF="[0.01 0.012 0 0 0 0  0.012 0.0144 0 0 0 0 1 1]"  LIM=[.075 .15 .15 .15]  Plot_On=off  MagdB_On=off  FreqRange=logspace(-2,2,500)
      settings: SourceProductName=Simscape Power Systems  SourceProductBaseCode=PS
  Multiport Switch1 : MultiPortSwitch  Inputs=4  InputSameDT=on
  PSS model3 : Constant  Value=0
  PSS model4 : Constant
  Pref : Constant
  Real-Imag to Complex : RealImagToComplex
  STG 023 : powerlib/Machines/Steam Turbine and Governor  gentype=Tandem-compound (single mass)  reg1="[ 1  0.05    0 ]"  reg2="[ 0.001  0.15 ]"  reg3="[ -0.1  0.1  0  4.496 ]"  N=3600  turb1="[ 0  10   3.3   0.5   ]"  turb2="[   0   0.36    0.36   0.28   ]"  HA="[ 0.046  1.430  1.465   0.192 ]"  KA="[ 90.44  53.88  64.59   62.94  ]"  DA="[ 0.0115  0.3575  0.3663   0.0137  ]"  ini1=0.95  ini2=[0.779316,-31.4247]
      settings: SourceProductName=Simscape Power Systems  SourceProductBaseCode=PS
  Sum2 : Sum  SaturateOnIntegerOverflow=on  InputSameDT=on  OutDataTypeStr=Inherit: Same as first input
  Sum3 : Sum  Inputs=-+  SaturateOnIntegerOverflow=on  InputSameDT=on  OutDataTypeStr=Inherit: Same as first input
  Terminator1 : Terminator
  Terminator2 : Terminator
  Terminator3 : Terminator
  Vref01 : Constant
  wref : Constant
  A : PMIOPort  Side=Left
  B : PMIOPort  Port=2  Side=Left
  C : PMIOPort  Port=3  Side=Left
  tag scope: EFD023=global, Pa023=global, Pe023=global, Pm023=global, Q023=global, Vt023=global, d_theta023=global, pss023=global, theta023=global, w023=global
  wires:
  Bus Selector1/7 -> Real-Imag to Complex/2  "<Stator voltage  vq (pu)>"
  Bus Selector1/6 -> Real-Imag to Complex/1  "<Stator voltage  vd (pu)>"
  wref/1 -> STG 023/1
  Vref01/1 -> AC4A Excitation System 02/1
  Bus Selector1/4 -> [d_theta023], STG 023/4  "<Rotor angle deviation  d_theta (rad)>"
  023/1 -> Bus Selector1/1, [M023]
  Bus Selector1/1 -> [w023], STG 023/3  "<Rotor speed  wm  (pu)>"
  Bus Selector1/3 -> "Delta w PSS (Kundur) 023 "/1, MB-PSS  023/1  "<Rotor speed deviation  dw (pu)>"
  Real-Imag to Complex/1 -> Complex to Magnitude-Angle/1
  Complex to Magnitude-Angle/1 -> AC4A Excitation System 02/2, [Vt023]
  AC4A Excitation System 02/1 -> 023/2, [EFD023]
  Multiport Switch1/1 -> AC4A Excitation System 02/4, [pss023]
  Bus Selector1/5 -> [theta023]  "<Rotor mechanical angle  theta (deg)>"
  Bus Selector1/2 -> [Pe023]  "<Output active power   Peo (pu)>"
  Bus Selector1/8 -> AC4A Excitation System 02/3  "<Field current  ifd (pu)>"
  STG 023/4 -> [Pm023], 023/1
  Pref/1 -> STG 023/2
  Bus Selector1/9 -> [Q023]  "<Output reactive power  Qeo (pu)>"
  PSS model4/1 -> Sum2/2
  Sum2/1 -> Multiport Switch1/1
  [PSSmodel] -> Sum2/1
  PSS model3/1 -> Multiport Switch1/2
  Sum3/1 -> [Pa023], "Delta Pa PSS 023 "/1  "Pm-Pe"
  "Delta Pa PSS 023 "/1 -> Multiport Switch1/5
  "Delta w PSS (Kundur) 023 "/1 -> Multiport Switch1/4
  [Pm023] -> Sum3/2
  [Pe023] -> Sum3/1
  MB-PSS  023/1 -> Multiport Switch1/3
  STG 023/1 -> Terminator3/1
  STG 023/2 -> Terminator1/1
  STG 023/3 -> Terminator2/1
  connections:
  023/RConn1 -- A/RConn1
  023/RConn2 -- B/RConn1
  023/RConn3 -- C/RConn1

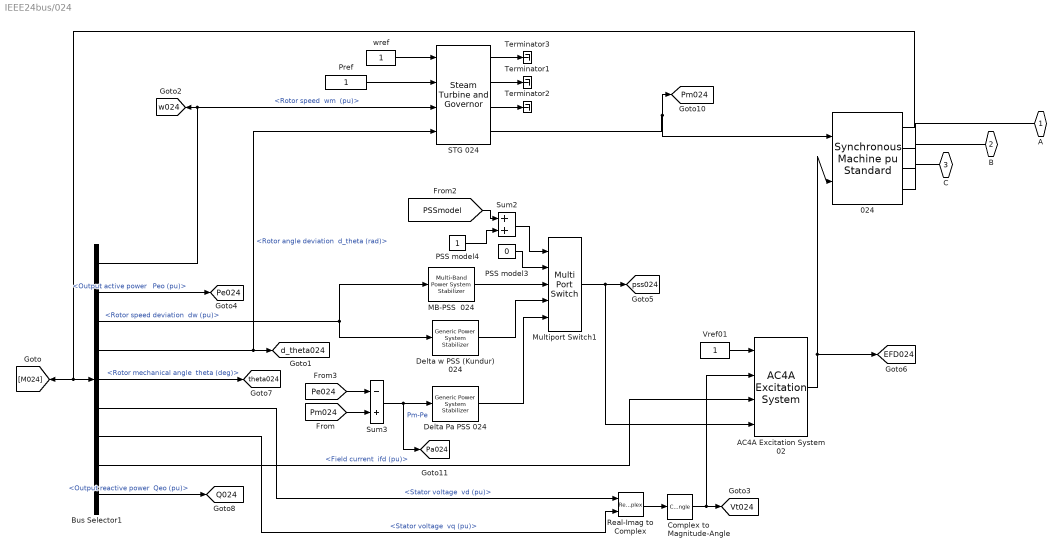
== system IEEE24bus/024 ==
  024 : powerlib/Machines/Synchronous Machine pu Standard  PresetModel=No  MechanicalLoad=Mechanical power Pm  ShowDetailedParameters=on  RotorType=Round  Units=per unit standard parameters  MeasurementBus=off  NominalParameters="[G_data(7,2)*1E6  G_data(7,3)*1E3  60]"  Reactances1=[G_data(7,6),G_data(7,8),G_data(7,10),G_data(7,7),G_data(7,12),G_data(7,14),G_data(7,5)]  Reactances2=[G_data(6,6),G_data(6,8),G_data(6,10),G_data(6,7),G_data(6,12),G_data(6,14),G_data(6,5)]  dAxisTimeConstants=Open-circuit  qAxisTimeConstants=Open-circuit  TimeConstants1="[G_data(6,9)  G_data(6,11)  G_data(6,13)  G_data(6,15)]"  TimeConstants2="[G_data(7,9)  G_data(7,11)  G_data(7,13)  G_data(7,15)]"  TimeConstants3="[  5.9  0.033  0.023  ]"  TimeConstants4=[ 8.0, 0.03, 0.3371, 0.0295 ]  TimeConstants5=[ 1.01, 0.053, 0.1 ]  TimeConstants6=[ 1.3201, 0.023, 1.0, 0.07 ]  TimeConstants7="[  1.01  0.053  0.051266  ]"  TimeConstants8=[ 1.3201, 0.0231, 0.3371, 0.0295 ]  StatorResistance=0  Mechanical="[ H024 0  4 ]"  PolePairs=4  InitialConditions=[0 -49.0871 0.832503 0.832503 0.832503 -10.6328 -130.633 109.367 2.39024]  SetSaturation=off  Saturation=[0.6404,0.7127,0.8441,0.9214,0.9956,1.082,1.19,1.316,1.457;0.7,0.7698,0.8872,0.9466,0.9969,1.046,1.1,1.151,1.201]  LoadFlowParameters=[1 3330000000 20000 0 0]  TsPowergui=0  TsBlock=-1  IterativeModel=Forward Euler  IterativeDiscreteModel=Trapezoidal non iterative  BusType=PV  Pref=G_data(7,2)*1e6  Qref=0  Qmin=-inf  Qmax=inf  PLF=0  QLF=0
      settings: SourceProductName=Simscape Power Systems
  AC4A Excitation System 02 : sps_avr/AC4A Excitation System  Tr=Exc(1,2)  KaTa="[Exc(1,3)   Exc(1,4)]"  VIminmax=[-10 10]  VRminmax=[-4.53 5.64]  TbTc="[Exc(1,5)  Exc(1,6)]"  Kc=0  v0=[1 2.3902]  TsBlock=0
      settings: SourceProductName=Simscape Power Systems  SourceProductBaseCode=PS
  Bus Selector1 : BusSelector  OutputSignals="Mechanical.Rotor speed  wm  (pu),Output active power   Peo (pu),Mechanical.Rotor speed deviation  dw (pu),Mechanical.Rotor angle deviation  d_theta (rad),Mechanical.Rotor mechanical angle  theta (deg),dq0 components.Stator voltage  vd (pu),dq0 components.Stator voltage  vq (pu),dq0 components.Field current  ifd (pu),Output reactive power  Qeo (pu)"
  Complex to Magnitude-Angle : ComplexToMagnitudeAngle  Output=Magnitude
  "Delta Pa PSS 024 " : powerlib/Machines/Generic Power System Stabilizer  Tsensor=15e-3  K=2.5*1.25  Twashout=1  Tleadlag1=[60e-3 1]  Tleadlag2=[0 0]  VSlimits=[-0.15 0.15]  Vinit=0  Plot_On=off  MagdB_On=on  FreqRange=logspace(-2,2,500)
      settings: SourceProductName=Simscape Power Systems  SourceProductBaseCode=PS
  "Delta w PSS (Kundur) 024 " : powerlib/Machines/Generic Power System Stabilizer  Tsensor=15e-3  K=30  Twashout=10  Tleadlag1=[50e-3 20e-3]  Tleadlag2=[3 5.4]  VSlimits=[-0.15 0.15]  Vinit=0  Plot_On=off  MagdB_On=on  FreqRange=logspace(-2,2,500)
      settings: SourceProductName=Simscape Power Systems  SourceProductBaseCode=PS
  MB-PSS  024 : powerlib/Machines/Multi-Band Power System Stabilizer  OperationMode=Simplified settings  Kg=1  GL=[0.1 10]  GI="[1  10]"  GH="[13  120]"  GLd=[66 66 9.4]  TcLF=[1.667 2 0 0 0 0 2 2.4 0 0 0 0 1 1]  GId=[66 66 47.6]  TcIF=[1 1 0.25 0.3 0 0 1 1 0.3 0.36 0 0 0 0]  GHd=[66 66 233]  TcHF="[0.01 0.012 0 0 0 0  0.012 0.0144 0 0 0 0 1 1]"  LIM=[.075 .15 .15 .15]  Plot_On=off  MagdB_On=off  FreqRange=logspace(-2,2,500)
      settings: SourceProductName=Simscape Power Systems  SourceProductBaseCode=PS
  Multiport Switch1 : MultiPortSwitch  Inputs=4  InputSameDT=on
  PSS model3 : Constant  Value=0
  PSS model4 : Constant
  Pref : Constant
  Real-Imag to Complex : RealImagToComplex
  STG 024 : powerlib/Machines/Steam Turbine and Governor  gentype=Tandem-compound (single mass)  reg1="[ 1  0.05    0 ]"  reg2="[ 0.001  0.15 ]"  reg3="[ -0.1  0.1  0  4.496 ]"  N=3600  turb1="[ 0  10   3.3   0.5   ]"  turb2="[   0   0.36    0.36   0.28   ]"  HA="[ 0.046  1.430  1.465   0.192 ]"  KA="[ 90.44  53.88  64.59   62.94  ]"  DA="[ 0.0115  0.3575  0.3663   0.0137  ]"  ini1=1  ini2=[0.779316,-31.4247]
      settings: SourceProductName=Simscape Power Systems  SourceProductBaseCode=PS
  Sum2 : Sum  SaturateOnIntegerOverflow=on  InputSameDT=on  OutDataTypeStr=Inherit: Same as first input
  Sum3 : Sum  Inputs=-+  SaturateOnIntegerOverflow=on  InputSameDT=on  OutDataTypeStr=Inherit: Same as first input
  Terminator1 : Terminator
  Terminator2 : Terminator
  Terminator3 : Terminator
  Vref01 : Constant
  wref : Constant
  A : PMIOPort  Side=Left
  B : PMIOPort  Port=2  Side=Left
  C : PMIOPort  Port=3  Side=Left
  tag scope: EFD024=global, Pa024=global, Pe024=global, Pm024=global, Q024=global, Vt024=global, d_theta024=global, pss024=global, theta024=global, w024=global
  wires:
  Bus Selector1/7 -> Real-Imag to Complex/2  "<Stator voltage  vq (pu)>"
  Bus Selector1/6 -> Real-Imag to Complex/1  "<Stator voltage  vd (pu)>"
  wref/1 -> STG 024/1
  Vref01/1 -> AC4A Excitation System 02/1
  Bus Selector1/4 -> [d_theta024], STG 024/4  "<Rotor angle deviation  d_theta (rad)>"
  024/1 -> Bus Selector1/1, [M024]
  Bus Selector1/1 -> [w024], STG 024/3  "<Rotor speed  wm  (pu)>"
  Bus Selector1/3 -> "Delta w PSS (Kundur) 024 "/1, MB-PSS  024/1  "<Rotor speed deviation  dw (pu)>"
  Real-Imag to Complex/1 -> Complex to Magnitude-Angle/1
  Complex to Magnitude-Angle/1 -> AC4A Excitation System 02/2, [Vt024]
  AC4A Excitation System 02/1 -> 024/2, [EFD024]
  Multiport Switch1/1 -> AC4A Excitation System 02/4, [pss024]
  Bus Selector1/5 -> [theta024]  "<Rotor mechanical angle  theta (deg)>"
  Bus Selector1/2 -> [Pe024]  "<Output active power   Peo (pu)>"
  Bus Selector1/8 -> AC4A Excitation System 02/3  "<Field current  ifd (pu)>"
  STG 024/4 -> [Pm024], 024/1
  Pref/1 -> STG 024/2
  Bus Selector1/9 -> [Q024]  "<Output reactive power  Qeo (pu)>"
  PSS model4/1 -> Sum2/2
  Sum2/1 -> Multiport Switch1/1
  [PSSmodel] -> Sum2/1
  PSS model3/1 -> Multiport Switch1/2
  Sum3/1 -> [Pa024], "Delta Pa PSS 024 "/1  "Pm-Pe"
  "Delta Pa PSS 024 "/1 -> Multiport Switch1/5
  "Delta w PSS (Kundur) 024 "/1 -> Multiport Switch1/4
  [Pm024] -> Sum3/2
  [Pe024] -> Sum3/1
  MB-PSS  024/1 -> Multiport Switch1/3
  STG 024/1 -> Terminator3/1
  STG 024/2 -> Terminator1/1
  STG 024/3 -> Terminator2/1
  connections:
  024/RConn1 -- A/RConn1
  024/RConn2 -- B/RConn1
  024/RConn3 -- C/RConn1
